simulink library "NSA_DEVS_LOGISTICS_SERVER"  (R2022b)
settings: Solver=VariableStepAuto  StartTime=0.0  StopTime=10.0  RelTol=1e-3
undefined symbols (not defined in the file or in its folder): add2, name
libraries: NSA_DEVS_MATH_OPERATIONS x1, NSA_DEVS_LOGISTICS_QUEUES x1, $bdroot x1, NSA_DEVS_SINKS x1
settings Model: Creator=david  LastModifiedBy=david

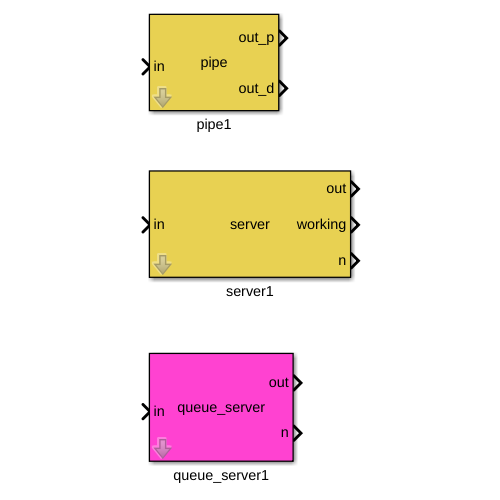
[thumbnail: Simulink's stored preview of the top-level diagram]
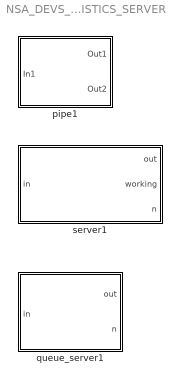
== system NSA_DEVS_LOGISTICS_SERVER ==
  pipe1 : Subsystem  mask{tau=[0,1], constructor='pipe("name",tau)'}
      mask Display:
      | disp("pipe");
      | 
      | port_label('input', 1, 'in');
      | port_label('output', 1, 'out_p');
      | port_label('output', 2, 'out_d');
  queue_server1 : Subsystem  mask{ts=1, tau=[0,1], tauOut=[0,1], debug=0, tw_name="varname", constructor='queue_server("name", ts, tau, tauOut, debug,tw_name)'}
      mask prompts: ts "service time"
      mask Display:
      | disp("queue_server");
      | 
      | port_label('input', 1, 'in');
      | port_label('output', 1, 'out');
      | port_label('output', 2, 'n');
  server1 : Subsystem  mask{ts=1.0, tau=[0,1], debug=0, constructor='server("name", ts, tau, debug)'}
      mask prompts: ts "service time"
      mask Display:
      | disp("server");
      | 
      | port_label('input', 1, 'in');
      | port_label('output', 1, 'out');
      | port_label('output', 2, 'working');
      | port_label('output', 3, 'n');

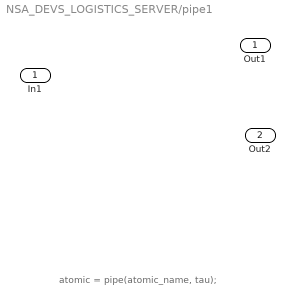
== system NSA_DEVS_LOGISTICS_SERVER/pipe1 ==
  note: atomic = pipe(atomic_name, tau);
  In1 : Inport
  Out1 : Outport
  Out2 : Outport  Port=2

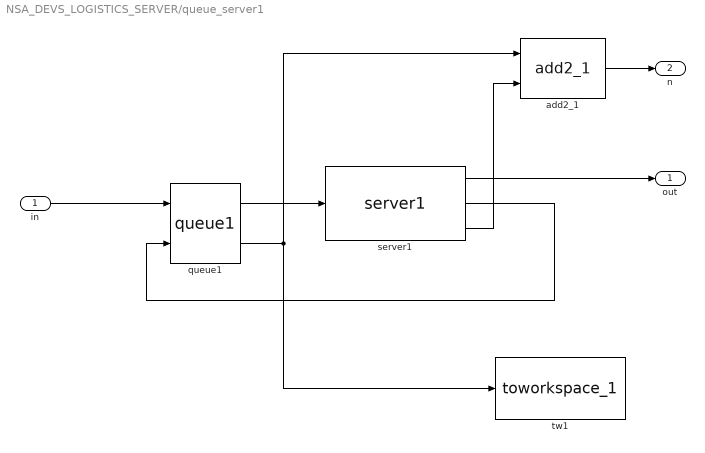
== system NSA_DEVS_LOGISTICS_SERVER/queue_server1 ==
  in : Inport
  add2_1 : NSA_DEVS_MATH_OPERATIONS/add2_1  tau=tau  debug=debug  constructor=add2(name, tau, debug)
      settings: SourceProductName=NSA_DEVS
  queue1 : NSA_DEVS_LOGISTICS_QUEUES/queue1  tau=3*tau  debug=debug  tD=3*tau  constructor=queue(name, tau, debug, tD)
      settings: LibrarySourceBlock=NSA_DEVS_LIB/queue1  SourceProductName=NSA_DEVS
  server1 : $bdroot/server1  ts=ts  tau=tau  debug=debug  constructor=server(name, tS, tau, debug)
      settings: LibrarySourceBlock=NSA_DEVS_LIB/server1
  tw1 : NSA_DEVS_SINKS/toworkspace_1  varname=tw_name  t0=0  tau=tauOut  format="\"'vector'\""  constructor="'toworkspace(\"name\",\"varname\",t0,tau,\"format\")'"
      settings: LibrarySourceBlock=NSA_DEVS_LIB/tw1  SourceProductName=NSA_DEVS
  out : Outport
  n : Outport  Port=2
  wires:
  in/1 -> queue1/1
  queue1/1 -> server1/1
  server1/1 -> out/1
  server1/2 -> queue1/2
  server1/3 -> add2_1/2
  queue1/2 -> add2_1/1, tw1/1
  add2_1/1 -> n/1

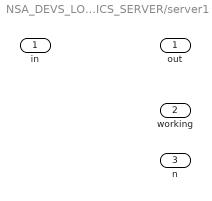
== system NSA_DEVS_LOGISTICS_SERVER/server1 ==
  in : Inport
  out : Outport
  working : Outport  Port=2
  n : Outport  Port=3
